simulink model "simcode"  (R2019b)
settings: Solver=VariableStepAuto  StartTime=0.0  StopTime=10.0  RelTol=1e-3
undefined symbols (not defined in the file): Ts_10kHz
libraries: dsparch4 x1
settings Model: Creator=Downstream  LastModifiedBy=Downstream

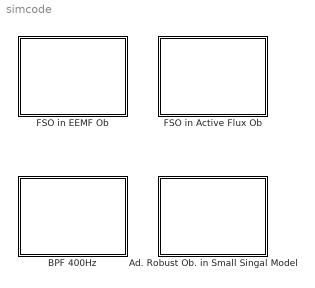
== system simcode ==
  Ad. Robust Ob. in Small Singal Model : Subsystem
  BPF 400Hz : Subsystem
  FSO in Active Flux Ob : Subsystem
  FSO in EEMF Ob : Subsystem

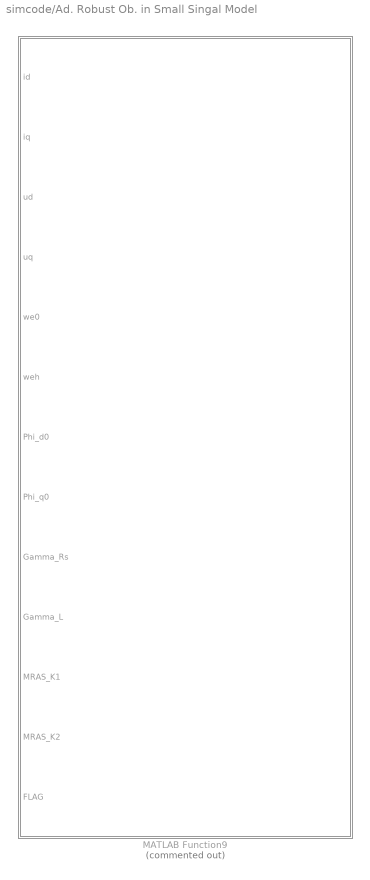
== system simcode/Ad. Robust Ob. in Small Singal Model ==
  MATLAB Function9 : MATLAB Function  Commented=on  TreatAsAtomicUnit=on

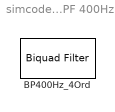
== system simcode/BPF 400Hz ==
  BP400Hz_4Ord : dsparch4/Biquad Filter  Tag=BlockMethodSubSystem  FilterSource=Dialog parameters  CoeffSource=Specify via dialog  FilterObject=BQF  IIRFiltStruct=Direct form II  BiQuadCoeffs=[1 0 -1 1 -1.93173306238314613 0.995528700328886185;1 0 -1 1 -1.93401211185528576 0.995605245274684303]  ScaleValues=[0.00313463184767947276;0.00313463184767947276;1]  IC=0  ICnum=0  ICden=0  a0Flag=Warning  optimizeScaleValues=on  ScaleValueMode=Specify via input port (g)  InputProcessing=Columns as channels (frame based)  roundingMode=Floor  overflowMode=off  scaleValueFracLength=14  denProdOutputFracLength=30  denAccumFracLength=30  secondMemoryFracLength=15
      settings: SourceProductName=DSP System Toolbox

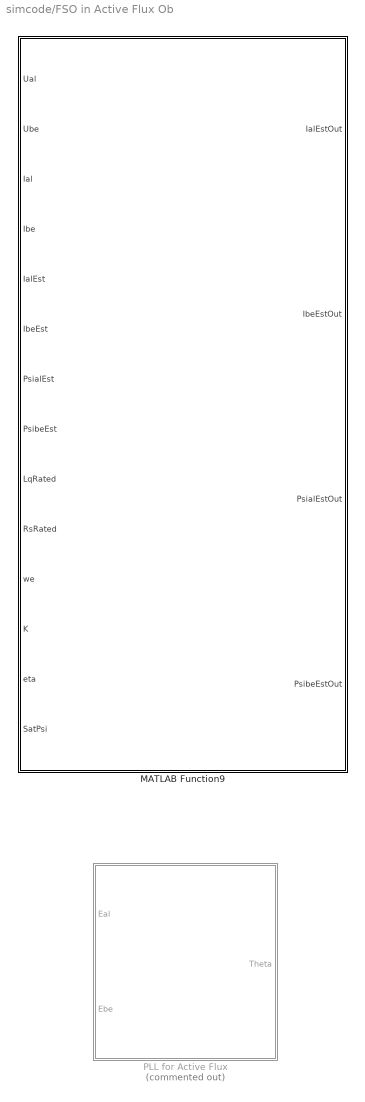
== system simcode/FSO in Active Flux Ob ==
  MATLAB Function9 : MATLAB Function  TreatAsAtomicUnit=on
  PLL for Active Flux : Subsystem  Commented=on

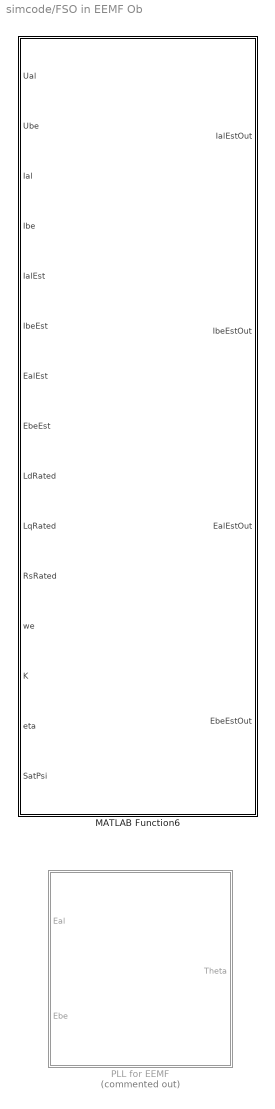
== system simcode/FSO in EEMF Ob ==
  MATLAB Function6 : MATLAB Function  TreatAsAtomicUnit=on
  PLL for EEMF : Subsystem  Commented=on

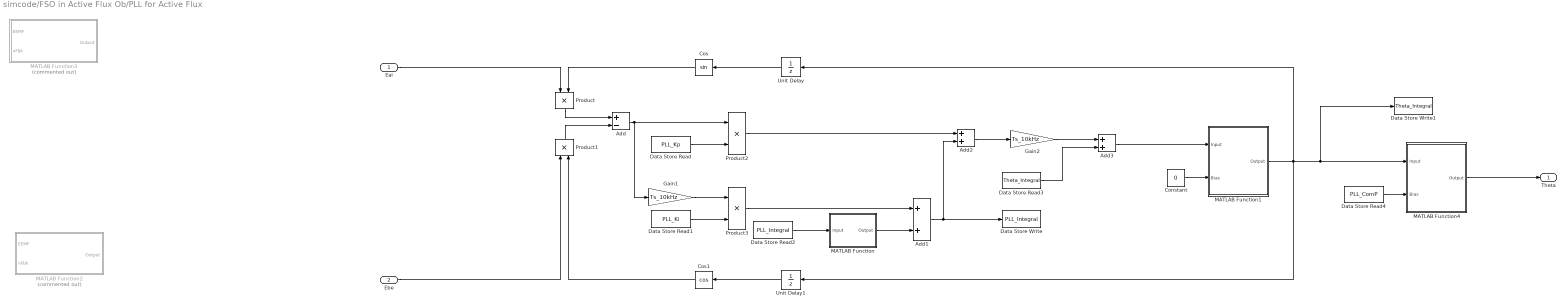
== system simcode/FSO in Active Flux Ob/PLL for Active Flux ==
  Eal : Inport
  Ebe : Inport  Port=2
  Add : Sum  Inputs=+-
  Add1 : Sum
  Add2 : Sum
  Add3 : Sum
  Constant : Constant  Value=0  SampleTime=-1
  Cos : Trigonometry  OutputSignalType=real
  Cos1 : Trigonometry  Operator=cos  OutputSignalType=real
  Data Store Read : DataStoreRead  DataStoreName=PLL_Kp
  Data Store Read1 : DataStoreRead  DataStoreName=PLL_Ki
  Data Store Read2 : DataStoreRead  DataStoreName=PLL_Integral
  Data Store Read3 : DataStoreRead  DataStoreName=Theta_Integral
  Data Store Read4 : DataStoreRead  DataStoreName=PLL_ComP
  Data Store Write : DataStoreWrite  DataStoreName=PLL_Integral
  Data Store Write1 : DataStoreWrite  DataStoreName=Theta_Integral
  Gain1 : Gain  Gain=Ts_10kHz
  Gain2 : Gain  Gain=Ts_10kHz
  MATLAB Function : MATLAB Function  TreatAsAtomicUnit=on
  MATLAB Function1 : MATLAB Function  TreatAsAtomicUnit=on
  MATLAB Function2 : MATLAB Function  Commented=on  TreatAsAtomicUnit=on
  MATLAB Function3 : MATLAB Function  Commented=on  TreatAsAtomicUnit=on
  MATLAB Function4 : MATLAB Function  TreatAsAtomicUnit=on
  Product{,1..3} (4 alike) : Product
  Unit Delay : UnitDelay  SampleTime=-1  HasFrameUpgradeWarning=on
  Unit Delay1 : UnitDelay  SampleTime=-1  HasFrameUpgradeWarning=on
  Theta : Outport
  wires:
  Eal/1 -> Product/1
  Ebe/1 -> Product1/1
  Product/1 -> Add/1
  Product1/1 -> Add/2
  Add/1 -> Gain1/1, Product2/1
  Data Store Read/1 -> Product2/2
  Data Store Read1/1 -> Product3/2
  Product3/1 -> Add1/1
  Data Store Read2/1 -> MATLAB Function/1(Input)
  Product2/1 -> Add2/1
  Gain1/1 -> Product3/1
  Add3/1 -> MATLAB Function1/1(Input)
  Cos/1 -> Product/2
  Cos1/1 -> Product1/2
  Add1/1 -> Add2/2, Data Store Write/1
  MATLAB Function/1(Output) -> Add1/2
  Add2/1 -> Gain2/1
  Data Store Read3/1 -> Add3/2
  Gain2/1 -> Add3/1
  Unit Delay/1 -> Cos/1
  Unit Delay1/1 -> Cos1/1
  Constant/1 -> MATLAB Function1/2(Bias)
  Data Store Read4/1 -> MATLAB Function4/2(Bias)
  MATLAB Function4/1(Output) -> Theta/1
  MATLAB Function1/1(Output) -> Data Store Write1/1, MATLAB Function4/1(Input), Unit Delay/1, Unit Delay1/1

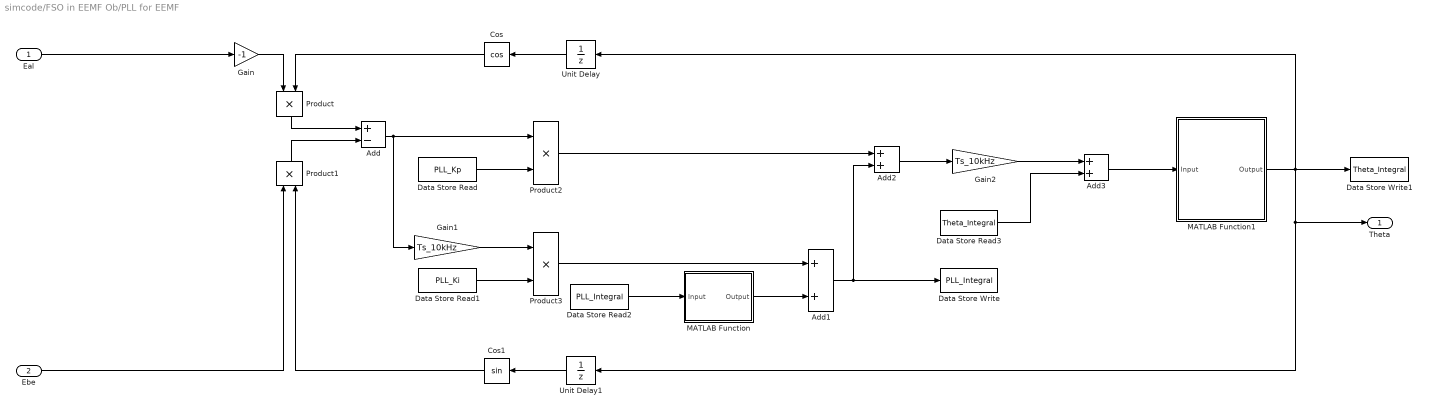
== system simcode/FSO in EEMF Ob/PLL for EEMF ==
  Eal : Inport
  Ebe : Inport  Port=2
  Add : Sum  Inputs=+-
  Add1 : Sum
  Add2 : Sum
  Add3 : Sum
  Cos : Trigonometry  Operator=cos  OutputSignalType=real
  Cos1 : Trigonometry  OutputSignalType=real
  Data Store Read : DataStoreRead  DataStoreName=PLL_Kp
  Data Store Read1 : DataStoreRead  DataStoreName=PLL_Ki
  Data Store Read2 : DataStoreRead  DataStoreName=PLL_Integral
  Data Store Read3 : DataStoreRead  DataStoreName=Theta_Integral
  Data Store Write : DataStoreWrite  DataStoreName=PLL_Integral
  Data Store Write1 : DataStoreWrite  DataStoreName=Theta_Integral
  Gain : Gain  Gain=-1
  Gain1 : Gain  Gain=Ts_10kHz
  Gain2 : Gain  Gain=Ts_10kHz
  MATLAB Function : MATLAB Function  TreatAsAtomicUnit=on
  MATLAB Function1 : MATLAB Function  TreatAsAtomicUnit=on
  Product{,1..3} (4 alike) : Product
  Unit Delay : UnitDelay  SampleTime=-1  HasFrameUpgradeWarning=on
  Unit Delay1 : UnitDelay  SampleTime=-1  HasFrameUpgradeWarning=on
  Theta : Outport
  wires:
  Eal/1 -> Gain/1
  Gain/1 -> Product/1
  Ebe/1 -> Product1/1
  Product/1 -> Add/1
  Product1/1 -> Add/2
  Add/1 -> Gain1/1, Product2/1
  Data Store Read/1 -> Product2/2
  Data Store Read1/1 -> Product3/2
  Product3/1 -> Add1/1
  Data Store Read2/1 -> MATLAB Function/1(Input)
  Product2/1 -> Add2/1
  Gain1/1 -> Product3/1
  Add3/1 -> MATLAB Function1/1(Input)
  Cos/1 -> Product/2
  Cos1/1 -> Product1/2
  Unit Delay/1 -> Cos/1
  Unit Delay1/1 -> Cos1/1
  Add1/1 -> Add2/2, Data Store Write/1
  MATLAB Function/1(Output) -> Add1/2
  Add2/1 -> Gain2/1
  Data Store Read3/1 -> Add3/2
  Gain2/1 -> Add3/1
  MATLAB Function1/1(Output) -> Unit Delay1/1, Theta/1, Data Store Write1/1, Unit Delay/1

== matlab function simcode/Ad. Robust Ob. in Small Singal Model/MATLAB Function9 ==
  data: id input; iq input; ud input; uq input; we0 input; weh input; Phi_d0 input; Phi_q0 input; Gamma_Rs input; Gamma_L input; MRAS_K1 input; MRAS_K2 input; FLAG input; MRAS_Rs data_store_memory; MRAS_Ld data_store_memory; MRAS_Lq data_store_memory; MRAS_idhat data_store_memory; MRAS_iqhat data_store_memory; MRAS_Ldq data_store_memory; MRAS_Init_Ldd data_store_memory; MRAS_Init_Ldq data_store_memory; MRAS_Init_Lqq data_store_memory; MRAS_Init_Rs data_store_memory
function MRAS_HOT(id,iq,ud,uq,we0,weh,Phi_d0,Phi_q0,Gamma_Rs,Gamma_L,MRAS_K1,MRAS_K2, FLAG)
global MRAS_Rs MRAS_Ld MRAS_Lq MRAS_Ldq MRAS_idhat MRAS_iqhat
global MRAS_Init_Rs MRAS_Init_Ldd MRAS_Init_Ldq MRAS_Init_Lqq
i = [id;iq];
u = [ud;uq];
i_hat = [MRAS_idhat;MRAS_iqhat];
L_hat = [MRAS_Ld MRAS_Ldq ; MRAS_Ldq MRAS_Lq];
J = [single(0) single(-1);single(1) single(0)];
I = [single(1) single(0);single(0) single(1) ];
i_tilde = i_hat - i;
i_sat = i_tilde;
for i = 1:2
    if(i_sat(i) > 0.01)
        i_sat(i) = 1;
    elseif(i_sat(i) < -0.01)
        i_sat(i) = -1;
    else
        i_sat(i) = i_sat(i) * single(100);
    end
end
Tsim = single(1e-4);
B = (L_hat^-1);
A = B * (-MRAS_Rs * I - we0 * J * L_hat);
% Phi = I + A * Tsim + single(0.5) * A^2 * Tsim^2;
% G   = Tsim * (I + single(0.5) * A * Tsim + single(0.167) * A^2 * Tsim^2) * B;

Phi = I + A * Tsim;
G   = Tsim * (I) * B;

dot_i_hat = A * i_hat + B * u - weh * B * J * [Phi_d0;Phi_q0];
i_hat_new = Phi * i_hat + G * (u - weh * J * [Phi_d0;Phi_q0] - MRAS_K1 * we0 * i_tilde - MRAS_K2 * i_sat);
for i = 1:2
    if(i_hat_new(i) > 10)
        i_hat_new(i) = 10;
    elseif(i_hat_new(i) < -10)
        i_hat_new(i) = -10;
    else
        i_hat_new(i) = i_hat_new(i);
    end
end

if(FLAG == uint16(0))
    dot_Rs_hat = Gamma_Rs * (i_tilde(1) * i_hat(1) + i_tilde(2) * i_hat(2));
%     dot_Rs_hat = Gamma_Rs * (i_tilde(1) * (i_hat(1) - weh/we0 * id0) + i_tilde(2) * (i_hat(2) - weh/we0 * iq0));
    dot_Ld_hat = Gamma_L * (( we0 * i_hat(1) * i_tilde(2) + dot_i_hat(1) * i_tilde(1))*single(1e-3));
    dot_Lq_hat = Gamma_L * ((-we0 * i_hat(2) * i_tilde(1) + dot_i_hat(2) * i_tilde(2))*single(1e-3)); 
    dot_Ldq_hat= Gamma_L * single(0.5) * (-we0 * i_hat(1) * i_tilde(1) + we0 * i_hat(2) * i_tilde(2) + dot_i_hat(2) * i_tilde(1) + dot_i_hat(1) * i_tilde(2)) * single(1e-3);
else
    dot_Rs_hat = single(0);
    dot_Ld_hat = single(0);
    dot_Lq_hat = single(0);
    dot_Ldq_hat= single(0);
    dot_i_hat = [single(0);single(0)];
    i_hat_new = [single(0);single(0)];
    MRAS_Rs = MRAS_Init_Rs;
    MRAS_Ld = MRAS_Init_Ldd;
    MRAS_Lq = MRAS_Init_Lqq;
    MRAS_Ldq = MRAS_Init_Ldq;
end
    MRAS_Rs = MRAS_Rs + dot_Rs_hat * Tsim;
    MRAS_Ld = MRAS_Ld + dot_Ld_hat * Tsim;
    MRAS_Lq = MRAS_Lq + dot_Lq_hat * Tsim;
    MRAS_Ldq= MRAS_Ldq+ dot_Ldq_hat* Tsim;
    if(MRAS_Rs < single(0))
        MRAS_Rs = single(0);
    elseif(MRAS_Rs > single(100))
        MRAS_Rs = single(100);
    end
    if(MRAS_Ld < single(0.1e-3))
        MRAS_Ld = single(0.1e-3);
    elseif(MRAS_Ld > single(500e-3))
        MRAS_Ld = single(500e-3);
    end
    if(MRAS_Lq < single(0.1e-3))
        MRAS_Lq = single(0.1e-3);
    elseif(MRAS_Lq > single(700e-3))
        MRAS_Lq = single(700e-3);
    end
	if(MRAS_Ldq < single(-100e-3))
        MRAS_Ldq = single(-100e-3);
	elseif(MRAS_Ldq > single(100e-3))
        MRAS_Ldq = single(100e-3);
	end
    MRAS_idhat = i_hat_new(1);
    MRAS_iqhat = i_hat_new(2);

== matlab function simcode/FSO in EEMF Ob/PLL for EEMF/MATLAB Function ==
  data: Input input; Output output
function Output = Saturation(Input)
Limit = single(2.1e3);
if(Input >= Limit)
    Output = Limit;
elseif(Input <= -Limit)
    Output = -Limit;
else
    Output = Input;
end

== matlab function simcode/FSO in EEMF Ob/PLL for EEMF/MATLAB Function1 ==
  data: Input input; Output output
function Output = Mod(Input)
Temp = Input;
if (Temp > single(2 * pi))
    Temp = Temp - 2 * pi;
elseif(Temp < 0)
    Temp = Temp + 2 * pi;
end
Output = Temp;

== matlab function simcode/FSO in EEMF Ob/MATLAB Function6 ==
  data: Ual input; IalEstOut output; Ube input; Ial input; Ibe input; IalEst input; IbeEst input; EalEst input; EbeEst input; LdRated input; LqRated input; RsRated input; we input; K input; eta input; SatPsi input; IbeEstOut output; EalEstOut output; EbeEstOut output
function [IalEstOut,IbeEstOut,EalEstOut,EbeEstOut] = FSO_EEMF(Ual,Ube,Ial,Ibe,IalEst,IbeEst,EalEst,EbeEst,LdRated,LqRated,RsRated,we,K,eta,SatPsi)
sign_al = IalEst - Ial;
sign_be = IbeEst - Ibe;
Ts = single(1e-4);

if(sign_al > single(SatPsi))
    sign_al = single(1);
elseif(sign_al < -single(SatPsi))
    sign_al = -single(1);
else
    sign_al = sign_al * single(1)/single(SatPsi);
end

if(sign_be > single(SatPsi))
    sign_be = single(1);
elseif(sign_be < -single(SatPsi))
    sign_be = -single(1);
else
    sign_be = sign_be * single(1)/single(SatPsi);
end
Temp1 = we * (LdRated - LqRated);
Temp2 = single(1) / LdRated;
% IalEstDot = single(1) / LdRated * (Ual - RsRated * IalEst - we * (LdRated - LqRated) * IbeEst - EalEst + K * sign_al);
% IbeEstDot = single(1) / LdRated * (Ube - RsRated * IbeEst + we * (LdRated - LqRated) * IalEst - EbeEst + K * sign_be);
%%report an error for code too long??
IalEstDot = Ual - RsRated * IalEst - Temp1 * IbeEst;
IalEstDot = IalEstDot - EalEst + K * sign_al;
IalEstDot = IalEstDot * Temp2;

IbeEstDot = Ube - RsRated * IbeEst + Temp1 * IalEst;
IbeEstDot = IbeEstDot - EbeEst + K * sign_be;
IbeEstDot = IbeEstDot * Temp2;

% T = K * [eta,we;-we,eta];
TempEal = eta * sign_al + we * sign_be;
TempEbe = -we  * sign_al + eta * sign_be;
EalEstDot =  - we * EbeEst + K * TempEal;
EbeEstDot =  we * EalEst + K * TempEbe;
% EalEstDot = - we * EbeEst + K * (eta * sign_al + we * sign_be);
% EbeEstDot =   we * EalEst + K * (-we  * sign_al + eta * sign_be);

IalEstOut = IalEst + IalEstDot * Ts;
IbeEstOut = IbeEst + IbeEstDot * Ts;

EalEstOut = EalEst + EalEstDot * Ts;
EbeEstOut = EbeEst + EbeEstDot * Ts;
end

== matlab function simcode/FSO in Active Flux Ob/MATLAB Function9 ==
  data: Ual input; IalEstOut output; Ube input; Ial input; Ibe input; IalEst input; IbeEst input; PsialEst input; PsibeEst input; LqRated input; RsRated input; we input; K input; eta input; SatPsi input; IbeEstOut output; PsialEstOut output; PsibeEstOut output
function [IalEstOut,IbeEstOut,PsialEstOut,PsibeEstOut] = FSO_ActiveFlux(Ual,Ube,Ial,Ibe,IalEst,IbeEst,PsialEst,PsibeEst,LqRated,RsRated,we,K,eta,SatPsi)
sign_al = IalEst - Ial;
sign_be = IbeEst - Ibe;
Ts = single(1e-4);

if(sign_al > single(SatPsi))
    sign_al = single(1);
elseif(sign_al < -single(SatPsi))
    sign_al = -single(1);
else
    sign_al = sign_al * single(1)/single(SatPsi);
end

if(sign_be > single(SatPsi))
    sign_be = single(1);
elseif(sign_be < -single(SatPsi))
    sign_be = -single(1);
else
    sign_be = sign_be * single(1)/single(SatPsi);
end
Temp1 = single(1) / LqRated;
% IalEstDot = single(1) / LqRated * (Ual - RsRated * IalEst - we * (-1) * PsibeEst + K * sign_al);
% IbeEstDot = single(1) / LqRated * (Ube - RsRated * IbeEst - we * PsialEst        + K * sign_be);
%%report an error for code too long??
IalEstDot = Ual - RsRated * IalEst;
IalEstDot = IalEstDot + we * PsibeEst + K * sign_al;
IalEstDot = IalEstDot * Temp1;

IbeEstDot = Ube - RsRated * IbeEst;
IbeEstDot = IbeEstDot - we * PsialEst + K * sign_be;
IbeEstDot = IbeEstDot * Temp1;

% T = h * I + eta * J; h = -K eta > 0
% T = -K * I + eta * J
TempEal =  -K * sign_al - eta * sign_be;
TempEbe = eta * sign_al - K * sign_be;
PsialEstDot =  - we * PsibeEst + TempEal;
PsibeEstDot =  we * PsialEst + TempEbe;
% EalEstDot = - we * EbeEst + K * (eta * sign_al + we * sign_be);
% EbeEstDot =   we * EalEst + K * (-we  * sign_al + eta * sign_be);

IalEstOut = IalEst + IalEstDot * Ts;
IbeEstOut = IbeEst + IbeEstDot * Ts;

PsialEstOut = PsialEst + PsialEstDot * Ts;
PsibeEstOut = PsibeEst + PsibeEstDot * Ts;
end

== matlab function simcode/FSO in Active Flux Ob/PLL for Active Flux/MATLAB Function ==
  data: Input input; Output output
function Output = Saturation(Input)
Limit = single(2.1e3);
if(Input >= Limit)
    Output = Limit;
elseif(Input <= -Limit)
    Output = -Limit;
else
    Output = Input;
end

== matlab function simcode/FSO in Active Flux Ob/PLL for Active Flux/MATLAB Function1 ==
  data: Input input; Output output; Bias input
function Output = Mod(Input,Bias)
Temp = Input + Bias;
if (Temp > single(2 * pi))
    Temp = Temp - 2 * pi;
elseif(Temp < 0)
    Temp = Temp + 2 * pi;
end
Output = Temp;

== matlab function simcode/FSO in Active Flux Ob/PLL for Active Flux/MATLAB Function2 ==
  data: EEMF input; Output output; nFbk input
function Output = SgnSpd(EEMF,nFbk)

Output = EEMF * single(sign(nFbk));

== matlab function simcode/FSO in Active Flux Ob/PLL for Active Flux/MATLAB Function3 ==
  data: EEMF input; Output output; nFbk input
function Output = SgnSpd(EEMF,nFbk)

Output = EEMF * single(sign(nFbk));

== matlab function simcode/FSO in Active Flux Ob/PLL for Active Flux/MATLAB Function4 ==
  data: Input input; Output output; Bias input
function Output = Mod(Input,Bias)
Temp = Input + Bias;
if (Temp > single(2 * pi))
    Temp = Temp - 2 * pi;
elseif(Temp < 0)
    Temp = Temp + 2 * pi;
end
Output = Temp;
